simulink model "Gaara"  (R2015a)
settings: Solver=ode23t  StartTime=0.0  StopTime=10.0  RelTol=1e-3
libraries: fl_lib x15, nesl_utility x4, elec_lib x1
settings Model: Creator=peer23peer  LastModifiedBy=peer23peer

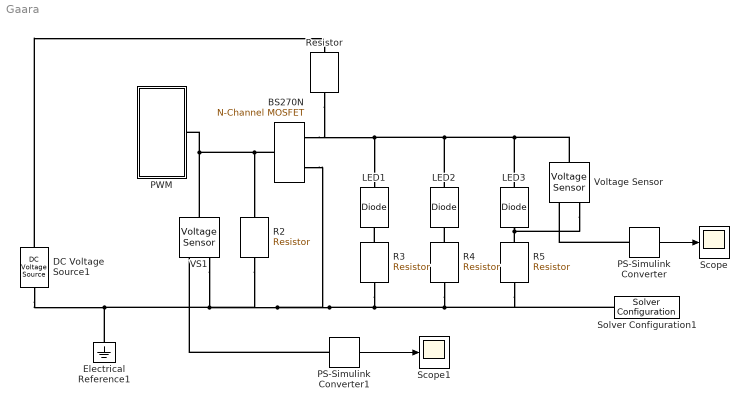
== system Gaara ==
  BS270N : elec_lib/Semiconductor Devices/N-Channel MOSFET  parameterization=1  prmDatasheet=2  prmEquCoeff=1  Beta=5 A/V^2  Rds=3.5 Ohm  Id=600 mA  Vgs=4.5 V  Vth=2.5 V  lam=0 1/V  Tmeas=25 C  RS=1e-4 Ohm  RD=0.01 Ohm  C_param=1  C_GS=270 pF  C_GD=80 pF  C_iss=50 pF  C_rss=5 pF  C_oss=25 pF  C_GS_vec=[ 270 300 290 280 295 255 ] pF  C_GD_vec=[ 450 400 300 190 95 55 ] pF  C_iss_vec=[ 720 700 590 470 390 310 ] pF  C_rss_vec=[ 450 400 300 190 95 55 ] pF  C_oss_vec=[ 900 810 690 420 270 170 ] pF  C_Vds_vec=[ 0.1 0.3 1 3 10 30 ] V  charge_linearity_param=1  C_OX=200 pF  V_C_OX=-0.5 V  dVth_dT=-6 mV/K  Rds_T2=3.5 Ohm  Tmeas2=125 C  BEXDatasheet=-1.5  BEXEquCoeff=-1.5  TdeviceDatasheet=25 C  TdeviceEquCoeff=25 C  Rth=[ 0 10 ] K/W  thermal_mass_parameterization=1  thermal_mass=[ 0 1 ] J/K  thermal_time_constant=[ 0 10 ] s  thermal_mass_initial_temperatures=[ 25 25 ] C
      settings: LogSimulationData=on
  DC Voltage Source1 : fl_lib/Electrical/Electrical Sources/DC Voltage Source  v0=5 V
  Electrical Reference1 : fl_lib/Electrical/Electrical Elements/Electrical Reference
  LED1 : fl_lib/Electrical/Electrical Elements/Diode  Vf=3.4 V  Ron=0.3 Ohm  Goff=1e-8 1/Ohm  i_specify=on  i_priority=High  i=600 mA  v_specify=off  v_priority=High  v=0 V
      settings: LogSimulationData=on
  LED2 : fl_lib/Electrical/Electrical Elements/Diode  Vf=3.4 V  Ron=0.3 Ohm  Goff=1e-8 1/Ohm  i_specify=on  i_priority=High  i=600 mA  v_specify=off  v_priority=High  v=0 V
      settings: LogSimulationData=on
  LED3 : fl_lib/Electrical/Electrical Elements/Diode  Vf=3.4 V  Ron=0.3 Ohm  Goff=1e-8 1/Ohm  i_specify=on  i_priority=High  i=600 mA  v_specify=off  v_priority=High  v=0 V
      settings: LogSimulationData=on
  PS-Simulink Converter : nesl_utility/PS-Simulink Converter  PhysicalDomain=network_engine_domain  SubClassName=ps_output  LeftPortType=input  RightPortType=output  PseudoPeriodic=off  Frequencies=[]  Unit=1  AffineConversion=off
  PS-Simulink Converter1 : nesl_utility/PS-Simulink Converter  PhysicalDomain=network_engine_domain  SubClassName=ps_output  LeftPortType=input  RightPortType=output  PseudoPeriodic=off  Frequencies=[]  Unit=1  AffineConversion=off
  PWM : Subsystem
  R2 : fl_lib/Electrical/Electrical Elements/Resistor  R=1 MOhm  i_specify=off  i_priority=High  i=0 A  v_specify=off  v_priority=High  v=0 V
  R3 : fl_lib/Electrical/Electrical Elements/Resistor  R=10 Ohm  i_specify=off  i_priority=High  i=0 A  v_specify=off  v_priority=High  v=0 V
  R4 : fl_lib/Electrical/Electrical Elements/Resistor  R=10 Ohm  i_specify=off  i_priority=High  i=0 A  v_specify=off  v_priority=High  v=0 V
  R5 : fl_lib/Electrical/Electrical Elements/Resistor  R=10 Ohm  i_specify=off  i_priority=High  i=0 A  v_specify=off  v_priority=High  v=0 V
  Resistor : fl_lib/Electrical/Electrical Elements/Resistor  R=500 Ohm  i_specify=off  i_priority=High  i=0 A  v_specify=off  v_priority=High  v=0 V
  Scope : Scope
      settings: TimeRange=10  YMin=0.25  YMax=3.5
  Scope1 : Scope
      settings: TimeRange=10  YMin=0.95  YMax=1.05
  Solver Configuration1 : nesl_utility/Solver Configuration  PhysicalDomain=network_engine_domain  SubClassName=solver  LeftPortType=input  RightPortType=generic  Accelerate=off  Tones=[]  Harmonics=[]  SimulateNoise=off  Profile=off  UseLocalSampling=off  EnableSwitchedLinearOptims=on  FrequencyDomain=off  UseCCode=off  RelTol=0.001  AbsTol=1e-06  MinStep=1e-09  ToWorkspace=off  RevertToSquareIcSolve=off  NumHomotopyIterations=100  DoDC=off  ResidualTolerance=1e-9  UseLocalSolver=on  LocalSolverChoice=NE_BACKWARD_EULER_ADVANCER  LocalSolverSampleTime=0.001  DoFixedCost=on  MaxNonlinIter=10  MaxModeIter=2  LinearAlgebra=Sparse  DelaysMemoryBudget=1024  AutomaticFiltering=on  FilteringTimeConstant=0.001
  VS1 : fl_lib/Electrical/Electrical Sensors/Voltage Sensor
  Voltage Sensor : fl_lib/Electrical/Electrical Sensors/Voltage Sensor
  wires:
  PS-Simulink Converter/1 -> Scope/1
  PS-Simulink Converter1/1 -> Scope1/1
  connections:
  BS270N/LConn1 -- VS1/LConn1 -- PWM/LConn1 -- R2/RConn1
  LED3/LConn1 -- LED2/LConn1 -- BS270N/RConn1 -- Resistor/RConn1 -- LED1/LConn1 -- Voltage Sensor/LConn1
  R3/LConn1 -- LED1/RConn1
  R4/LConn1 -- LED2/RConn1
  R5/LConn1 -- Voltage Sensor/RConn2 -- LED3/RConn1
  Electrical Reference1/LConn1 -- R2/LConn1 -- Solver Configuration1/RConn1 -- R5/RConn1 -- R4/RConn1 -- R3/RConn1 -- BS270N/RConn2 -- VS1/RConn2 -- DC Voltage Source1/RConn1
  PS-Simulink Converter/LConn1 -- Voltage Sensor/RConn1
  DC Voltage Source1/LConn1 -- Resistor/LConn1
  PS-Simulink Converter1/LConn1 -- VS1/RConn1

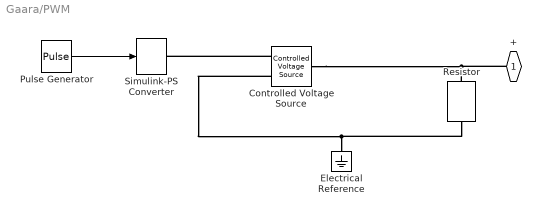
== system Gaara/PWM ==
  Controlled Voltage Source : fl_lib/Electrical/Electrical Sources/Controlled Voltage Source
  Electrical Reference : fl_lib/Electrical/Electrical Elements/Electrical Reference
  Pulse Generator : DiscretePulseGenerator  PulseType=Time based  Amplitude=3.3  Period=1/1000  PulseWidth=50
  Resistor : fl_lib/Electrical/Electrical Elements/Resistor  R=22 kOhm  i_specify=off  i_priority=High  i=0 A  v_specify=off  v_priority=High  v=0 V
  Simulink-PS Converter : nesl_utility/Simulink-PS Converter  PhysicalDomain=network_engine_domain  SubClassName=ps_input  LeftPortType=input  RightPortType=output  PseudoPeriodic=off  Frequencies=[]  NoiseDistribution=none  NoiseParameters=[]  Unit=1  AffineConversion=off  InputFiltering=off  SimscapeFilterOrder=1  InputFilterTimeConstant=0.001  UdotUserProvided=1
  + : PMIOPort  Port=1  Side=Left
  wires:
  Pulse Generator/1 -> Simulink-PS Converter/1
  connections:
  Controlled Voltage Source/RConn1 -- Simulink-PS Converter/RConn1
  Controlled Voltage Source/RConn2 -- Resistor/RConn1 -- Electrical Reference/LConn1
  +/RConn1 -- Controlled Voltage Source/LConn1 -- Resistor/LConn1
